simulink model "player"  (Simulink 8.6)
settings: Solver=FixedStepDiscrete  StartTime=0.0  StopTime=inf  FixedStep=Ts  RelTol=1e-3
InitFcn:
  | init;
libraries: WBToolboxLibrary x5
settings Model: Creator=makaveli  LastModifiedBy=makaveli
settings DataIOCC: SaveFormat=Dataset  SignalLoggingSaveFormat=Dataset
settings OptimizationCC: ExpressionDepthLimit=128
settings DebuggingCC: UnderspecifiedInitializationDetection=Simplified  MergeDetectMultiDrivingBlocksExec=error  SolverPrmCheckMsg=none  FcnCallInpInsideContextMsg=EnableAllAsError  StateNameClashWarn=none
settings HardwareCC: ProdBitPerPointer=64  ProdLargestAtomicFloat=Float  ProdIntDivRoundTo=Zero  ProdEndianess=LittleEndian  ProdWordSize=64  ProdHWDeviceType=Intel->x86-64 (Windows64)
settings GRTTargetCC: GeneratePreprocessorConditionals=Use local settings  CombineOutputUpdateFcns=on  GRTInterface=off
settings ConfigComp: CovModelRefEnable=off

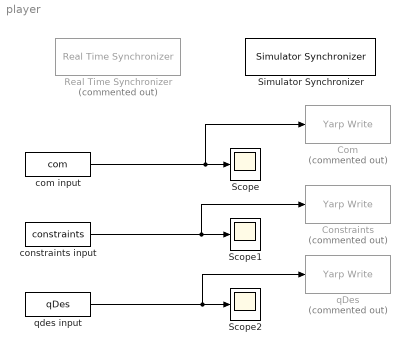
== system player ==
  Com : WBToolboxLibrary/Utilities/Yarp Write  Commented=on  portName=comPort  autoconnect=on  errorOnConnection=on
  Constraints : WBToolboxLibrary/Utilities/Yarp Write  Commented=on  portName=constraintsPort  autoconnect=on  errorOnConnection=on
  Real Time Synchronizer : WBToolboxLibrary/Utilities/Real Time Synchronizer  Commented=on  period=Ts
  Scope : Scope
  Scope1 : Scope
  Scope2 : Scope
  Simulator Synchronizer : WBToolboxLibrary/Utilities/Simulator Synchronizer  period=Ts  serverPortName='/clock/rpc'  clientPortName='/WBT_synchronizer/rpc:o'
  com input : FromWorkspace  VariableName=com  SampleTime=0
  constraints input : FromWorkspace  VariableName=constraints  SampleTime=0
  qDes : WBToolboxLibrary/Utilities/Yarp Write  Commented=on  portName=qDesPort  autoconnect=on  errorOnConnection=on
  qdes input : FromWorkspace  VariableName=qDes  SampleTime=0
  wires:
  com input/1 -> Com/1, Scope/1
  constraints input/1 -> Constraints/1, Scope1/1
  qdes input/1 -> qDes/1, Scope2/1
